simulink model "untitled"  (R2020a)
settings: Solver=FixedStepAuto  StartTime=0.0  StopTime=10.0  FixedStep=0.001  RelTol=1e-3
undefined symbols (not defined in the file): T, Tdia
libraries: simulink x1
settings Model: Creator=sebastian  LastModifiedBy=sebastian

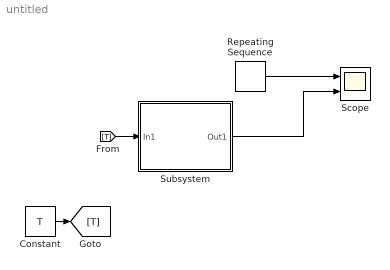
== system untitled ==
  Constant : Constant  Value=T
  Repeating Sequence : simulink/Sources/Repeating Sequence  rep_seq_t=[0 Tdia Tdia+0.001 T]  rep_seq_y=[0 0 1 1]
  Scope : Scope  NumInputPorts=2
  Subsystem : Subsystem
  wires:
  Repeating Sequence/1 -> Scope/1
  Constant/1 -> [T]
  [T] -> Subsystem/1(In1)
  Subsystem/1(Out1) -> Scope/2

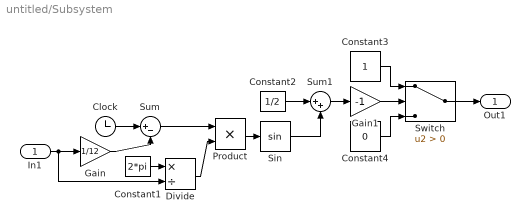
== system untitled/Subsystem ==
  In1 : Inport
  Clock : Clock
  Constant1 : Constant  Value=2*pi
  Constant2 : Constant  Value=1/2
  Constant3 : Constant
  Constant4 : Constant  Value=0
  Divide : Product  Inputs=*/
  Gain : Gain  Gain=1/12
  Gain1 : Gain  Gain=-1
  Product : Product
  Sin : Trigonometry
  Sum : Sum  Inputs=|+-
  Sum1 : Sum  Inputs=|++
  Switch : Switch  Criteria=u2 > Threshold
  Out1 : Outport
  wires:
  Constant1/1 -> Divide/1
  Divide/1 -> Product/2
  Constant2/1 -> Sum1/1
  Sum/1 -> Product/1
  Gain/1 -> Sum/2
  Constant3/1 -> Switch/1
  Sum1/1 -> Gain1/1
  Sin/1 -> Sum1/2
  Constant4/1 -> Switch/3
  Gain1/1 -> Switch/2
  Product/1 -> Sin/1
  In1/1 -> Divide/2, Gain/1
  Clock/1 -> Sum/1
  Switch/1 -> Out1/1
